simulink model "AM_Modulation"  (R2024b)
settings: Solver=VariableStepAuto  StartTime=0.0  StopTime=2/3400  RelTol=1e-3

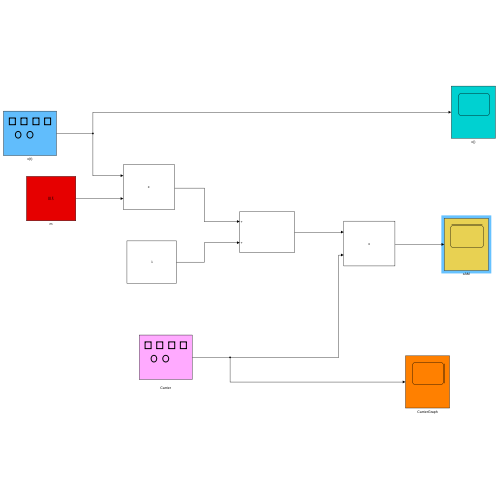
[thumbnail: Simulink's stored preview of the top-level diagram]
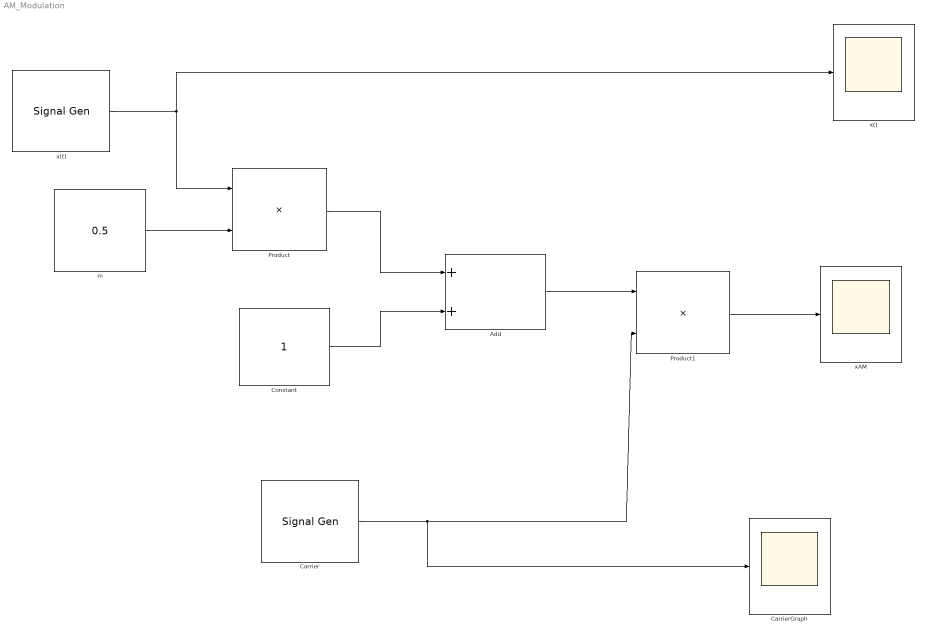
== system AM_Modulation ==
  " Carrier" : SignalGenerator  Amplitude=10  Frequency=15*10000
  Add : Sum
  CarrierGraph : Scope
  Constant : Constant
  Product : Product
  Product1 : Product
  m : Constant  Value=0.5
  x() : Scope
  x(t) : SignalGenerator  Amplitude=2  Frequency=5000
  xAM : Scope
  wires:
  x(t)/1 -> x()/1, Product/1
  m/1 -> Product/2
  Constant/1 -> Add/2
  Product/1 -> Add/1
  Add/1 -> Product1/1
  " Carrier"/1 -> Product1/2, CarrierGraph/1
  Product1/1 -> xAM/1
